simulink model "KeyControlaMIL"  (R2020b)
settings: Solver=FixedStepAuto  StartTime=0.0  StopTime=60  FixedStep=5  RelTol=1e-3
undefined symbols (not defined in the file or in its folder): sigbuilder_block
settings Model: Creator=99003745  LastModifiedBy=99003745

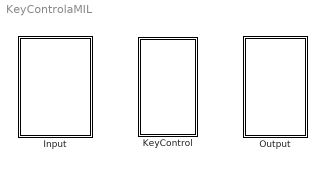
== system KeyControlaMIL ==
  Input : Subsystem
  KeyControl : Subsystem
  Output : Subsystem

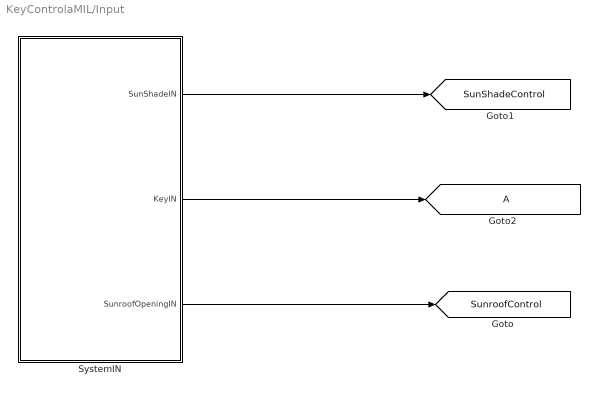
== system KeyControlaMIL/Input ==
  SystemIN : Subsystem  Tag=STV Subsys  LoadFcn=sigbuilder_block('load');  StartFcn=sigbuilder_block('start');  StopFcn=sigbuilder_block('stop');  ClipboardFcn=sigbuilder_block('clipboard');  mask(Sigbuilder block){tuvar=[0:10]}
      mask help: Simulink:masks:SigbuilderBlock_MD
      mask init:
      | if ~strcmp(get_param(bdroot(gcbh),'SimulationStatus'),'stopped') tuvar = sigbuilder_block('maskInit'); end
      settings: CopyFcn=sigbuilder_block('copy');  DeleteFcn=sigbuilder_block('delete');  ModelCloseFcn=sigbuilder_block('modelClose');  PreSaveFcn=sigbuilder_block('preSave');  PauseFcn=sigbuilder_block('pause');  ContinueFcn=sigbuilder_block('continue');  NameChangeFcn=sigbuilder_block('namechange');  OpenFcn=sigbuilder_block('open',[558.75 205.5 550.5 399.75 ]);  CloseFcn=sigbuilder_block('close');
      mask Display: plot(0, 0, 100, 100,[2, 2, 32, 32, 2], [68, 8, 8, 68, 68],[32, 2], [38, 38], [32, 19, 2],[53, 60, 44], [32, 17, 17, 2],[16, 16, 31, 31]);txt = getActiveGroup(gcbh);text(2, 100, txt,'verticalAlignment', 'top');
  tag scope: A=global, SunShadeControl=global, SunroofControl=global
  wires:
  SystemIN/2(KeyIN) -> [A]
  SystemIN/1(SunShadeIN) -> [SunShadeControl]
  SystemIN/3(SunroofOpeningIN) -> [SunroofControl]

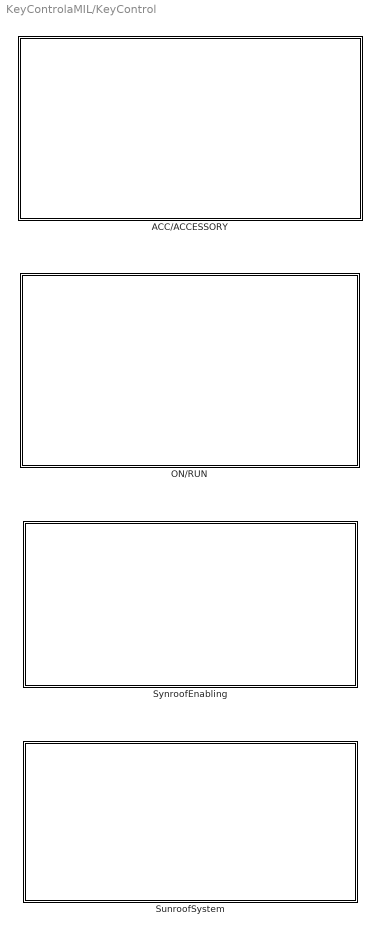
== system KeyControlaMIL/KeyControl ==
  ACC/ACCESSORY : Subsystem
  ON/RUN : Subsystem
  SunroofSystem : Subsystem
  SynroofEnabling : Subsystem

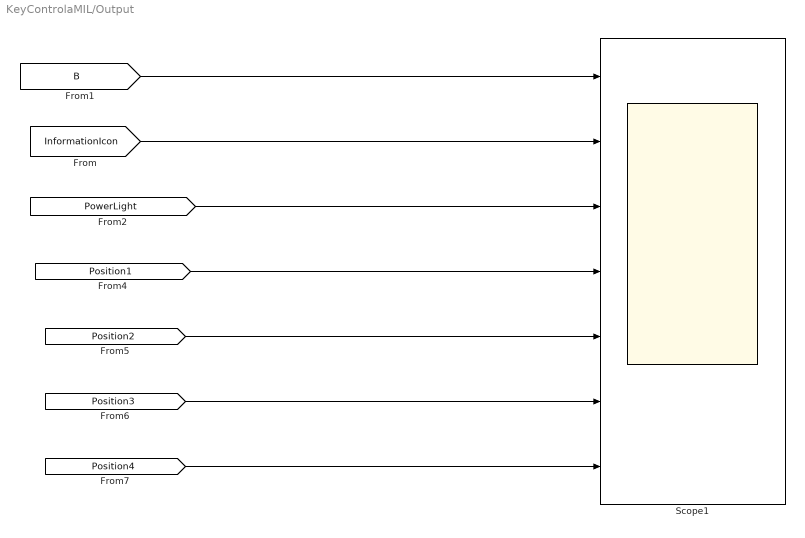
== system KeyControlaMIL/Output ==
  Scope1 : Scope  NumInputPorts=7
  wires:
  [B] -> Scope1/1
  [PowerLight] -> Scope1/3
  [Position1] -> Scope1/4
  [Position2] -> Scope1/5
  [Position3] -> Scope1/6
  [Position4] -> Scope1/7
  [InformationIcon] -> Scope1/2

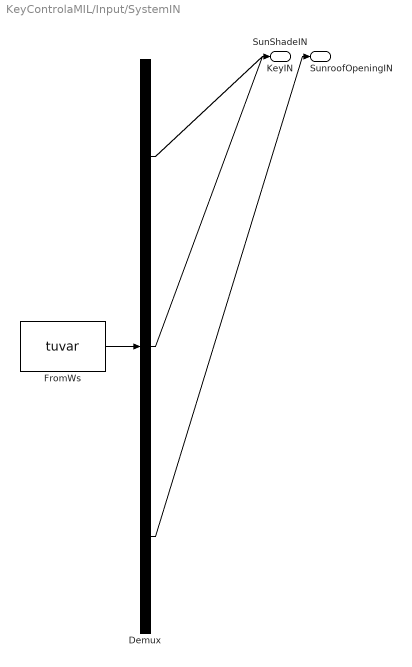
== system KeyControlaMIL/Input/SystemIN ==
  Demux : Demux  Tag=STV Demux  Outputs=3
      settings: DisplayOption=none
  FromWs : FromWorkspace  Tag=STV FromWs  VariableName=tuvar
      SigBuilderData=|
      | common.afterFinalStr = 'Extrapolate'
      | common.sampleTime = 0
      | dataSet.timeRange = [0 10]
      | dataSet.name = 'Group 1'
      | sbobj.Groups.Name = 'Group 1'
      | sbobj.Groups.Signals(1).Name = 'SunShadeIN'
      | sbobj.Groups.Signals(1).XData = [0 2 4 6 8 10 12 14 16 18 20 22 24 26 28 30 32 34 36 38 40 42 44 46 48 50 52 54 56 58 60]
      | sbobj.Groups.Signals(1).YData = [0 0 0 0 0 -0.05 1 1 1 1 1 1 1 1 1 1 1 1 0 0 0 1 1 1 1 1 0 0 0 0 0]
      | sbobj.Groups.Signals(2).Name = 'KeyIN'
      | sbobj.Groups.Signals(2).XData = [0 2 4 6 8 10 12 14 16 18 20 22 24 26 28 30 32 34 36 38 40 42 44 46 48 50 52 54 56 58 60]
      | sbobj.Groups.Signals(2).YData = [0 0 0 0 1 1 1 1 2 2 2 2 3 3 3 3 2 2 2 2 1 1 1 1 0 0 0 0 0 1 1]
      | sbobj.Groups.Signals(3).Name = 'SunroofOpeningIN'
      | sbobj.Groups.Signals(3).XData = [0 2 4 6 8 10 12 14 16 18 20 22 24 26 28 30 32 34 36 38 40 42 44 46 48 50 52 54 56 58 60]
      | sbobj.Groups.Signals(3).YData = [0 10 20 30 40 50 60 70 80 90 100 90 80 70 60 50 40 30 20 10 0 10 20 30 40 50 60 70 80 90 100]
      | sbobj.Groups.TimeRange = [0 60]
  SunShadeIN : Outport  Tag=STV Outport
  KeyIN : Outport  Tag=STV Outport  Port=2
  SunroofOpeningIN : Outport  Tag=STV Outport  Port=3
  wires:
  FromWs/1 -> Demux/1
  Demux/1 -> SunShadeIN/1
  Demux/2 -> KeyIN/1
  Demux/3 -> SunroofOpeningIN/1

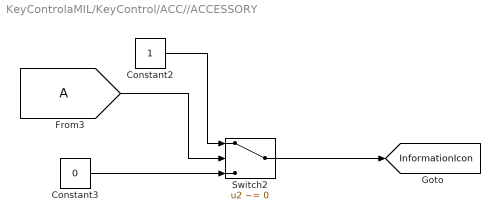
== system KeyControlaMIL/KeyControl/ACC//ACCESSORY ==
  Constant2 : Constant
  Constant3 : Constant  Value=0
  Switch2 : Switch  Criteria=u2 ~= 0
  tag scope: InformationIcon=global
  wires:
  Switch2/1 -> [InformationIcon]
  [A] -> Switch2/2
  Constant3/1 -> Switch2/3
  Constant2/1 -> Switch2/1

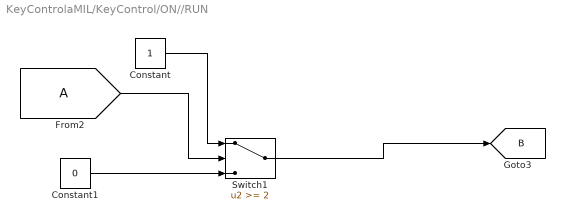
== system KeyControlaMIL/KeyControl/ON//RUN ==
  Constant : Constant
  Constant1 : Constant  Value=0
  Switch1 : Switch  Threshold=2
  tag scope: B=global
  wires:
  [A] -> Switch1/2
  Switch1/1 -> [B]
  Constant/1 -> Switch1/1
  Constant1/1 -> Switch1/3

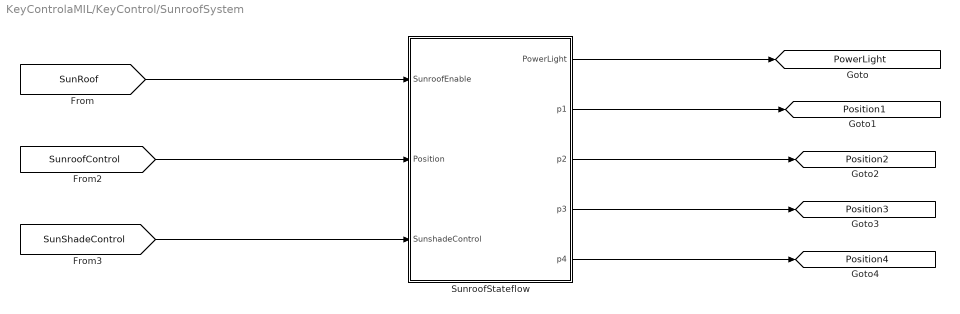
== system KeyControlaMIL/KeyControl/SunroofSystem ==
  SunroofStateflow : Stateflow chart  TreatAsAtomicUnit=on
  tag scope: Position1=global, Position2=global, Position3=global, Position4=global, PowerLight=global
  wires:
  [SunroofControl] -> SunroofStateflow/2(Position)
  SunroofStateflow/5(p4) -> [Position4]
  [SunRoof] -> SunroofStateflow/1(SunroofEnable)
  [SunShadeControl] -> SunroofStateflow/3(SunshadeControl)
  SunroofStateflow/3(p2) -> [Position2]
  SunroofStateflow/4(p3) -> [Position3]
  SunroofStateflow/1(PowerLight) -> [PowerLight]
  SunroofStateflow/2(p1) -> [Position1]

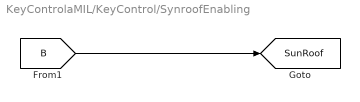
== system KeyControlaMIL/KeyControl/SynroofEnabling ==
  tag scope: SunRoof=global
  wires:
  [B] -> [SunRoof]

== stateflow chart KeyControlaMIL/KeyControl/SunroofSystem/SunroofStateflow ==
  state SunshadeOff
    entry:
    PowerLight=0;
  state SunshadeOn
    entry:
    PowerLight=1;
  state SunroofEnable
    entry:
    PowerLight=2;
    p1=0;
    p2=0;
    p3=0;
    p4=0;
  state P4
    entry:
    p1=1;
    p2=1;
    p3=1;
    p4=1;
  state P3
    entry:
    p1=1;
    p2=1;
    p3=1;
    p4=0;
  state P2
    entry:
    p1=1;
    p2=1;
    p3=0;
    p4=0;
  state P1
    entry:
    p1=1;
    p2=0;
    p3=0;
    p4=0;
  (default) -> SunshadeOff
  SunshadeOff -> SunshadeOn : [SunshadeControl==1]
  SunshadeOn -> SunshadeOff [order 2] : [SunshadeControl==0]
  SunroofEnable -> SunshadeOn [order 1] : [SunroofEnable==0]
  SunshadeOn -> SunroofEnable [order 1] : [SunshadeControl==1&&SunroofEnable==1]
  P4 -> SunroofEnable [order 2] : [SunshadeControl==0&&SunroofEnable==0]
  SunroofEnable -> P3 [order 4] : [SunshadeControl==1&&SunroofEnable==1 && Position>=50 && Position<=75]
  SunroofEnable -> P4 [order 3] : [SunshadeControl==1&&SunroofEnable==1 && Position>75 && Position<=100]
  SunroofEnable -> P1 [order 2] : [SunshadeControl==1&&SunroofEnable==1 && Position>0 && Position<=25]
  P3 -> SunroofEnable [order 3] : [SunshadeControl==0&&SunroofEnable==0]
  P1 -> SunroofEnable [order 2] : [SunshadeControl==0&&SunroofEnable==0 && Position>=0 && Position<50]
  P2 -> SunroofEnable [order 3] : [SunshadeControl==0&&SunroofEnable==0]
  SunroofEnable -> P2 [order 5] : [SunshadeControl==1&&SunroofEnable==1 && Position>=25 && Position<50]
  P1 -> P2 [order 1] : [SunshadeControl==1&&SunroofEnable==1 && Position>=25 && Position<50]
  P2 -> P3 [order 1] : [SunshadeControl==1&&SunroofEnable==1 && Position>=50 && Position<75]
  P3 -> P4 [order 1] : [SunshadeControl==1&&SunroofEnable==1 && Position>=75 && Position<100]
  P2 -> P1 [order 2] : [SunshadeControl==1&&SunroofEnable==1 && Position>0 && Position<=25]
  P3 -> P2 [order 2] : [SunshadeControl==1&&SunroofEnable==1 && Position>25&& Position<=50]
  P4 -> P3 [order 1] : [SunshadeControl==1&&SunroofEnable==1 && Position>50 && Position<=75]
  data: SunroofEnable input; Position input; SunshadeControl input; PowerLight output; p1 output; p2 output; p3 output; p4 output
